simulink model "Propeller_Control_Prime_Mover"  (R2021b)
settings: Solver=VariableStepAuto  StartTime=0.0  StopTime=30.0  RelTol=1e-3
libraries: fl_lib x11, nesl_utility x4, slpidlib x2, ee_lib x1, sdl_lib x1
settings Model: Creator=Rishi  LastModifiedBy=Rishi

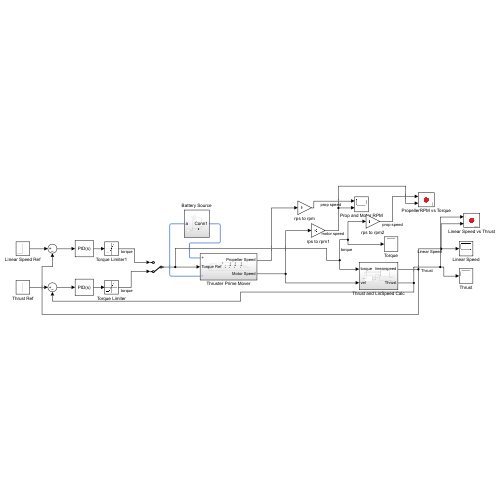
[thumbnail: Simulink's stored preview of the top-level diagram]
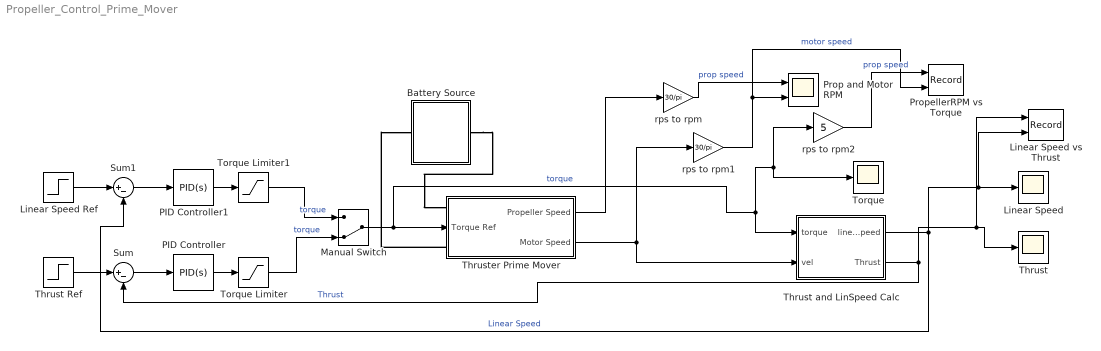
== system Propeller_Control_Prime_Mover ==
  Battery Source : Subsystem
  Linear Speed : Scope
  Linear Speed Ref : Step  After=3  SampleTime=0
  Linear Speed vs Thrust : Record  FileSettingsInternal="{\"entries\":[{\"content\":{\"excelSettings\":{\"content\":{},\"type\":\"Streamout.ExcelSettings\"}},\"type\":\"Streamout.FileSettingStorage\",\"uuid\":\"f38cdbd6-b5c5-4525-af82-986570d2f1bb\"}],\"packageUris\":[\"http://schema.mathworks.com/mf0/streamout_blocks/R2020a\"],\"version\":\"1.0\"}"  Layout=[1 1]  SignalsInternal="{\"entries\":[{\"content\":{\"signals\":[{\"content\":{\"blockPath\":[\"Propeller_Control_Prime_Mover/Linear Speed vs Thrust\"],\"channel\":[],\"dimensions\":[1],\"domain\":\"Propeller_Control_Prime_Mover/Linear Speed vs Thrust\",\"lineColor\":\"#a2142f\",\"plots\":[1],\"port\":1,\"sid\":[\"\"],\"signalID\":332,\"signalName\":\"Thrust\"},\"type\":\"RecordBlkView.Signal\",\"uuid\":\"575c3137-ab97-410f-b3d3-826d395c1239\"},{\"content\":{\"blockPath\":[\"Propeller_Control_Prime_Mover/Linear Speed vs Thrust\"],\"channel\":[],\"dimensions\":[1],\"domain\":\"Propeller_Control_Prime_Mover/Linear Speed vs Thrust\",\"lineColor\":\"#139fff\",\"plots\":[1],\"port\":2,\"sid\":[\"\"],\"signalID\":336,\"signalName\":\"Linear Speed\"},\"type\":\"RecordBlkView.Signal\",\"uuid\":\"f93925d7-110e-4419-9b3e-40073e6103b4\"}]},\"type\":\"RecordBlkView.InputSignals\",\"uuid\":\"601741f8-a10c-45ed-a42c-22fcf3854612\"}],\"packageUris\":[\"http://schema.mathworks.com/mf0/streamout_blocks/R2020a\"],\"version\":\"1.0\"}"  VisualizationBindings="{\"xyplotplugin\":{\"info\":[{\"series\":[{\"bindingParametersList\":[{\"parameter\":\"X-Axis\",\"signalID\":332,\"signalName\":\"Thrust\"},{\"parameter\":\"Y-Axis\",\"signalID\":336,\"signalName\":\"Linear Speed\"}],\"seriesID\":64183}],\"subplotID\":1}]}}"  CompatibilityTag=XY
  Manual Switch : ManualSwitch  CurrentSetting=0
  PID Controller : slpidlib/PID Controller  Controller=PID  Form=Parallel  TimeDomain=Continuous-time  UseExternalTs=off  SampleTime=-1  IntegratorMethod=Forward Euler  FilterMethod=Forward Euler  ControllerParametersSource=internal  P=0.0808899689686358  I=0.058736929683079  D=-0.00606531904447916  UseFilter=on  N=1.40895966466238  TunerSelectOption=Transfer Function Based (PID Tuner App)  InitialConditionSource=internal  InitialConditionForIntegrator=0  InitialConditionForFilter=0  DifferentiatorICPrevScaledInput=0  ExternalReset=none  TrackingMode=off  Kt=1  LimitOutput=off  SatLimitsSource=internal  UpperSaturationLimit=inf  LowerSaturationLimit=-inf  LinearizeAsGain=on  AntiWindupMode=none  Kb=1  POutMin=[]  POutMax=[]  IOutMin=[]  IOutMax=[]  DOutMin=[]  DOutMax=[]  NOutMin=[]  NOutMax=[]  SumOutMin=[]  SumOutMax=[]  SaturationOutMin=[]  SaturationOutMax=[]  PParamMin=[]  PParamMax=[]  IParamMin=[]  IParamMax=[]  DParamMin=[]  DParamMax=[]  NParamMin=[]  NParamMax=[]  KbParamMin=[]  KbParamMax=[]  KtParamMin=[]  KtParamMax=[]  KbOutMin=[]  KbOutMax=[]  KtOutMin=[]  KtOutMax=[]  IntegratorOutMin=[]  IntegratorOutMax=[]  FilterOutMin=[]  FilterOutMax=[]  SumI1OutMin=[]  SumI1OutMax=[]  SumI2OutMin=[]  SumI2OutMax=[]  SumI3OutMin=[]  SumI3OutMax=[]  SumI4OutMin=[]  SumI4OutMax=[]  SumDOutMin=[]  SumDOutMax=[]  DifferentiatorOutMin=[]  DifferentiatorOutMax=[]  FilterDiffOutCoefMin=[]  FilterDiffOutCoefMax=[]  ReciprocalOutMin=[]  ReciprocalOutMax=[]  SumDenOutMin=[]  SumDenOutMax=[]  SumNumOutMin=[]  SumNumOutMax=[]  DivideOutMin=[]  DivideOutMax=[]  UdiffTsProdOutMin=[]  UdiffTsProdOutMax=[]  NTsProdOutMin=[]  NTsProdOutMax=[]  UintegralTsProdOutMin=[]  UintegralTsProdOutMax=[]  UngainTsProdOutMin=[]  UngainTsProdOutMax=[]  IntegratorContinuousStateAttributes=''  IntegratorStateMustResolveToSignalObject=off  IntegratorRTWStateStorageClass=Auto  FilterContinuousStateAttributes=''  FilterStateMustResolveToSignalObject=off  FilterRTWStateStorageClass=Auto  ParallelPVariant=InternalParameters  IdealPVariant=Disabled  IVariant=InternalParameters  DVariant=InternalParameters  IntegratorVariant=Continuous  SatVariant=Disabled  AWVariant=Passthrough  PCopyVariant=Disabled  TRVariant=Disabled  FdbkBlocksVariant=Forward  IdealPFdbkVariant=Disabled  SatFdbkVariant=Disabled  DerivativeFilterVariant=ContFilter  NVariant=InternalParameters  NCopyVariant=Disabled  FilterICVariant=InternalICsFilter  IntegratorICVariant=InternalICs  ExternalResetVariant=Disabled  TRSumVariant=Passthrough  SumFdbkVariant=Disabled  SumVariant=Sum_PID  TsampFilterVariant=InternalTs  TsampNgainVariant=Passthrough  TsampIntegralVariant=Passthrough  ExternalSaturationOutDataTypeStr=Inherit: Same as second input
  PID Controller1 : slpidlib/PID Controller  Controller=PID  Form=Parallel  TimeDomain=Continuous-time  UseExternalTs=off  SampleTime=-1  IntegratorMethod=Forward Euler  FilterMethod=Forward Euler  ControllerParametersSource=internal  P=0  I=0.957539779346888  D=0  UseFilter=on  N=100  TunerSelectOption=Transfer Function Based (PID Tuner App)  InitialConditionSource=internal  InitialConditionForIntegrator=0  InitialConditionForFilter=0  DifferentiatorICPrevScaledInput=0  ExternalReset=none  TrackingMode=off  Kt=1  LimitOutput=off  SatLimitsSource=internal  UpperSaturationLimit=inf  LowerSaturationLimit=-inf  LinearizeAsGain=on  AntiWindupMode=none  Kb=1  POutMin=[]  POutMax=[]  IOutMin=[]  IOutMax=[]  DOutMin=[]  DOutMax=[]  NOutMin=[]  NOutMax=[]  SumOutMin=[]  SumOutMax=[]  SaturationOutMin=[]  SaturationOutMax=[]  PParamMin=[]  PParamMax=[]  IParamMin=[]  IParamMax=[]  DParamMin=[]  DParamMax=[]  NParamMin=[]  NParamMax=[]  KbParamMin=[]  KbParamMax=[]  KtParamMin=[]  KtParamMax=[]  KbOutMin=[]  KbOutMax=[]  KtOutMin=[]  KtOutMax=[]  IntegratorOutMin=[]  IntegratorOutMax=[]  FilterOutMin=[]  FilterOutMax=[]  SumI1OutMin=[]  SumI1OutMax=[]  SumI2OutMin=[]  SumI2OutMax=[]  SumI3OutMin=[]  SumI3OutMax=[]  SumI4OutMin=[]  SumI4OutMax=[]  SumDOutMin=[]  SumDOutMax=[]  DifferentiatorOutMin=[]  DifferentiatorOutMax=[]  FilterDiffOutCoefMin=[]  FilterDiffOutCoefMax=[]  ReciprocalOutMin=[]  ReciprocalOutMax=[]  SumDenOutMin=[]  SumDenOutMax=[]  SumNumOutMin=[]  SumNumOutMax=[]  DivideOutMin=[]  DivideOutMax=[]  UdiffTsProdOutMin=[]  UdiffTsProdOutMax=[]  NTsProdOutMin=[]  NTsProdOutMax=[]  UintegralTsProdOutMin=[]  UintegralTsProdOutMax=[]  UngainTsProdOutMin=[]  UngainTsProdOutMax=[]  IntegratorContinuousStateAttributes=''  IntegratorStateMustResolveToSignalObject=off  IntegratorRTWStateStorageClass=Auto  FilterContinuousStateAttributes=''  FilterStateMustResolveToSignalObject=off  FilterRTWStateStorageClass=Auto  ParallelPVariant=InternalParameters  IdealPVariant=Disabled  IVariant=InternalParameters  DVariant=InternalParameters  IntegratorVariant=Continuous  SatVariant=Disabled  AWVariant=Passthrough  PCopyVariant=Disabled  TRVariant=Disabled  FdbkBlocksVariant=Forward  IdealPFdbkVariant=Disabled  SatFdbkVariant=Disabled  DerivativeFilterVariant=ContFilter  NVariant=InternalParameters  NCopyVariant=Disabled  FilterICVariant=InternalICsFilter  IntegratorICVariant=InternalICs  ExternalResetVariant=Disabled  TRSumVariant=Passthrough  SumFdbkVariant=Disabled  SumVariant=Sum_PID  TsampFilterVariant=InternalTs  TsampNgainVariant=Passthrough  TsampIntegralVariant=Passthrough  ExternalSaturationOutDataTypeStr=Inherit: Same as second input
  Prop and Motor RPM : Scope  NumInputPorts=2
  PropellerRPM vs Torque : Record  FileSettingsInternal="{\"entries\":[{\"content\":{\"excelSettings\":{\"content\":{},\"type\":\"Streamout.ExcelSettings\"}},\"type\":\"Streamout.FileSettingStorage\",\"uuid\":\"e7f1eaa3-e328-4bb8-9999-0087dc1a7fd9\"}],\"packageUris\":[\"http://schema.mathworks.com/mf0/streamout_blocks/R2020a\"],\"version\":\"1.0\"}"  Layout=[1 1]  SignalsInternal="{\"entries\":[{\"content\":{\"signals\":[{\"content\":{\"blockPath\":[\"Propeller_Control_Prime_Mover/PropellerRPM vs Torque\"],\"channel\":[],\"dimensions\":[1],\"domain\":\"Propeller_Control_Prime_Mover/PropellerRPM vs Torque\",\"lineColor\":\"#64d413\",\"plots\":[],\"port\":1,\"sid\":[\"\"],\"signalID\":340,\"signalName\":\"prop speed\"},\"type\":\"RecordBlkView.Signal\",\"uuid\":\"83d94086-b276-4ada-afda-b43e66d6f884\"},{\"content\":{\"blockPath\":[\"Propeller_Control_Prime_Mover/PropellerRPM vs Torque\"],\"channel\":[],\"dimensions\":[1],\"domain\":\"Propeller_Control_Prime_Mover/PropellerRPM vs Torque\",\"lineColor\":\"#ff13a6\",\"plots\":[],\"port\":2,\"sid\":[\"\"],\"signalID\":344,\"signalName\":\"motor speed\"},\"type\":\"RecordBlkView.Signal\",\"uuid\":\"5dc8b065-5f7c-49e4-81b4-50af2d2f00db\"}]},\"type\":\"RecordBlkView.InputSignals\",\"uuid\":\"fe2e9c10-fa43-4037-ab47-88955eef5109\"}],\"packageUris\":[\"http://schema.mathworks.com/mf0/streamout_blocks/R2020a\"],\"version\":\"1.0\"}"  VisualizationBindings="{\"xyplotplugin\":{\"info\":[{\"series\":[{\"bindingParametersList\":[{\"parameter\":\"X-Axis\",\"signalID\":9,\"signalName\":\"prop speed\"},{\"parameter\":\"Y-Axis\",\"signalID\":12,\"signalName\":\"motor speed\"}],\"seriesID\":39395}],\"subplotID\":1}]}}"  CompatibilityTag=XY
  Sum : Sum  Inputs=|+-
  Sum1 : Sum  Inputs=|+-
  Thrust : Scope
  Thrust Ref : Step  After=98  SampleTime=0
  Thrust and LinSpeed Calc : Subsystem
  Thruster Prime Mover : Subsystem
      settings: PortSchema="{\"entries\":[{\"content\":{\"sides\":[{\"content\":{\"connectorIds\":[\"LConn1\",\"In1\",\"LConn2\"]},\"type\":\"ConnectorPlacement.EquallySpacedRectSide\",\"uuid\":\"b491ab2f-3c91-4c99-a87c-c51358079dd3\"},{\"content\":{\"connectorIds\":[\"Out1\",\"Out2\"],\"side\":\"RIGHT\"},\"type\":\"ConnectorPlacement.EquallySpacedRectSide\",\"uuid\":\"68efad03-1b86-4427-b220-44990910d7ff\"},{\"content\":{\"connectorIds\":[],\"side\":\"TOP\"},\"type\":\"ConnectorPlacement.EquallySpacedRectSide\",\"uuid\":\"6c75a4a0-8522-4b4f-a5fb-dcf7bbf55362\"}]},\"type\":\"ConnectorPlacement.EquallySpacedConnector\",\"uuid\":\"388c7d20-d64b-442d-a00b-569f4554c2be\"}],\"packageUris\":[\"http://schema.mathworks.com/mf0/Connector/R2020b\"],\"version\":\"1.0\"}"
  Torque : Scope
  Torque Limiter : Saturate  UpperLimit=5  LowerLimit=0
  Torque Limiter1 : Saturate  UpperLimit=5  LowerLimit=0
  rps to rpm : Gain  Gain=30/pi
  rps to rpm1 : Gain  Gain=30/pi
  rps to rpm2 : Gain  Gain=5
  wires:
  Thrust Ref/1 -> Sum/1
  Thruster Prime Mover/2(Motor Speed) -> rps to rpm1/1, Thrust and LinSpeed Calc/2(vel)
  Torque Limiter/1 -> Manual Switch/2  "torque"
  PID Controller/1 -> Torque Limiter/1
  Sum/1 -> PID Controller/1
  Thruster Prime Mover/1(Propeller Speed) -> rps to rpm/1
  Torque Limiter1/1 -> Manual Switch/1  "torque"
  PID Controller1/1 -> Torque Limiter1/1
  Linear Speed Ref/1 -> Sum1/1
  Sum1/1 -> PID Controller1/1
  Manual Switch/1 -> rps to rpm2/1, Torque/1, Thrust and LinSpeed Calc/1(torque), Thruster Prime Mover/1(Torque Ref)  "torque"
  Thrust and LinSpeed Calc/2(Thrust) -> Linear Speed vs Thrust/1, Thrust/1, Sum/2  "Thrust"
  Thrust and LinSpeed Calc/1(linearspeed) -> Linear Speed vs Thrust/2, Linear Speed/1, Sum1/2  "Linear Speed"
  rps to rpm/1 -> Prop and Motor RPM/1  "prop speed"
  rps to rpm1/1 -> PropellerRPM vs Torque/2, Prop and Motor RPM/2  "motor speed"
  rps to rpm2/1 -> PropellerRPM vs Torque/1  "prop speed"
  connections:
  Battery Source/LConn1 -- Thruster Prime Mover/LConn1
  Thruster Prime Mover/LConn2 -- Battery Source/RConn1

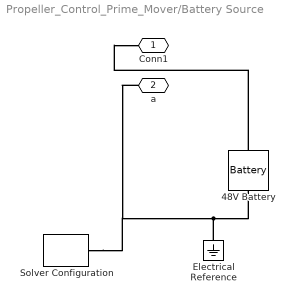
== system Propeller_Control_Prime_Mover/Battery Source ==
  48V Battery : ee_lib/Sources/Battery  Vnom=48 V  prm_dir=1  R1_dis=2 Ohm  R1_ch=2 Ohm  R1=2 Ohm  prm_AH=1  AH=50 A*hr  V1=11.5 V  AH1=25 A*hr  prm_R2=1  R2=2000 Ohm  prm_dyn=1  Rp1=0.005 Ohm  tau1=30 s  Rp2=0.005 Ohm  tau2=30 s  Rp3=0.005 Ohm  tau3=30 s  Rp4=0.005 Ohm  tau4=30 s  Rp5=0.005 Ohm  tau5=30 s  prm_fade=1  N_fade=100  AH_fade=45 A*hr  R1_fade=2.02 Ohm  R1_ch_fade=2.02 Ohm  V1_fade=10.35 V  prm_age=1  prm_age_OCV=1  OCV_age=0.9  SOC_age=60  delta_time_age_vec=[0] d  temperature_age_vec=[273] K  OCV_scaling_age=2.2134e6  OCV_offset_age=1.632e6  temp_exp_age=0.515833569 V  t_exp_age=0.75  i_specify=off  i_priority=None  i=0 A  i_nominal_specify=off  i_nominal_unit=A  i_nominal_value=1  v_specify=off  v_priority=None  v=0 V  v_nominal_specify=off  v_nominal_unit=V  v_nominal_value=1  charge_specify=off  charge_priority=High  charge=50 A*hr  charge_nominal_specify=off  charge_nominal_unit=A*hr  charge_nominal_value=1  num_cycles_specify=off  num_cycles_priority=High  num_cycles=0  num_cycles_nominal_specify=off  num_cycles_nominal_unit=1  num_cycles_nominal_value=1  Tmeas=298.15 K  Tmeas_age=298.15 K  Vnom_T2=12 V  R1_T2=2.2 Ohm  R1_T2_dis=2.2 Ohm  R1_T2_ch=2.2 Ohm  V1_T2=11.4 V  R2_T2=2200 Ohm  Rp1_T2=0.005 Ohm  tau1_T2=30 s  Rp2_T2=0.005 Ohm  tau2_T2=30 s  Rp3_T2=0.005 Ohm  tau3_T2=30 s  Rp4_T2=0.005 Ohm  tau4_T2=30 s  Rp5_T2=0.005 Ohm  tau5_T2=30 s  Tmeas2=273.15 K  thermal_mass=30000 J/K  temperature_specify=off  temperature_priority=High  temperature=298.15 K  temperature_nominal_specify=off  temperature_nominal_unit=K  temperature_nominal_value=1
  Electrical Reference : fl_lib/Electrical/Electrical Elements/Electrical Reference
  Solver Configuration : nesl_utility/Solver Configuration  PhysicalDomain=network_engine_domain  SubClassName=solver  LeftPortType=input  RightPortType=generic  Tones=[]  Harmonics=[]  SimulateNoise=off  Profile=off  UseLocalSampling=off  EnableSwitchedLinearOptims=on  FrequencyDomain=off  UseCCode=off  RelTol=0.001  AbsTol=1e-06  MinStep=1e-09  ToWorkspace=off  RevertToSquareIcSolve=off  NumHomotopyIterations=100  PhasorMode=off  PhasorModeNumHarmonics=1  DoDC=off  ResidualTolerance=1e-09  UseLocalSolver=off  LocalSolverChoice=NE_BACKWARD_EULER_ADVANCER  LocalSolverSampleTime=0.001  DoFixedCost=off  MaxNonlinIter=3  MaxModeIter=2  ComputeImpulses=off  ImpulseIterations=2  LinearAlgebra=auto  EquationFormulation=NE_TIME_EF  DelaysMemoryBudget=1024  AutomaticFiltering=on  FilteringTimeConstant=0.001  PartitionStorageMethod=AS_NEEDED  PartitionMemoryBudget=1024  PartitionMethod=ROBUST
      settings: SourceProductBaseCode=PW,SS
  Conn1 : PMIOPort  Side=Left
  a : PMIOPort  Port=2  Side=Right
  connections:
  Electrical Reference/LConn1 -- 48V Battery/RConn1 -- a/RConn1 -- Solver Configuration/RConn1
  48V Battery/LConn1 -- Conn1/RConn1

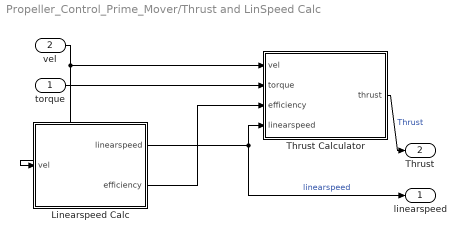
== system Propeller_Control_Prime_Mover/Thrust and LinSpeed Calc ==
  torque : Inport
  vel : Inport  Port=2
  Linearspeed Calc : MATLAB Function  TreatAsAtomicUnit=on
  Thrust Calculator : MATLAB Function  TreatAsAtomicUnit=on
  linearspeed : Outport
  Thrust : Outport  Port=2
  wires:
  vel/1 -> Linearspeed Calc/1(vel), Thrust Calculator/1(vel)
  torque/1 -> Thrust Calculator/2(torque)
  Thrust Calculator/1(thrust) -> Thrust/1  "Thrust"
  Linearspeed Calc/1(linearspeed) -> linearspeed/1, Thrust Calculator/4(linearspeed)  "linearspeed"
  Linearspeed Calc/2(efficiency) -> Thrust Calculator/3(efficiency)

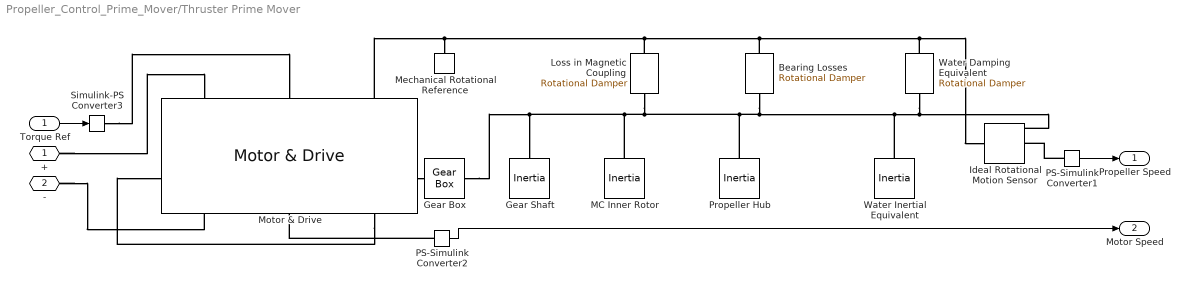
== system Propeller_Control_Prime_Mover/Thruster Prime Mover ==
  Torque Ref : Inport
  Bearing Losses : fl_lib/Mechanical/Rotational Elements/Rotational Damper  D=0.01 N*m/(rad/s)  w_specify=off  w_priority=None  w=0 rad/s  w_nominal_specify=off  w_nominal_unit=rad/s  w_nominal_value=1  t_specify=off  t_priority=None  t=0 N*m  t_nominal_specify=off  t_nominal_unit=N*m  t_nominal_value=1
  Gear Box : fl_lib/Mechanical/Mechanisms/Gear Box  ratio=5  t_in_specify=off  t_in_priority=None  t_in=0 N*m  t_in_nominal_specify=off  t_in_nominal_unit=N*m  t_in_nominal_value=1  t_out_specify=off  t_out_priority=None  t_out=0 N*m  t_out_nominal_specify=off  t_out_nominal_unit=N*m  t_out_nominal_value=1
  Gear Shaft : fl_lib/Mechanical/Rotational Elements/Inertia  inertia=6.525e-08 kg*m^2  num_ports=foundation.enum.numPorts2.one  w_specify=off  w_priority=High  w=0 rad/s  w_nominal_specify=off  w_nominal_unit=rad/s  w_nominal_value=1  t_specify=off  t_priority=None  t=0 N*m  t_nominal_specify=off  t_nominal_unit=N*m  t_nominal_value=1
  Ideal Rotational Motion Sensor : fl_lib/Mechanical/Mechanical Sensors/Ideal Rotational Motion Sensor  wrap_angle=simscape.enum.onoff.off  offset=0 rad
  Loss in Magnetic Coupling : fl_lib/Mechanical/Rotational Elements/Rotational Damper  D=0.001 N*m*s/rad  w_specify=off  w_priority=None  w=0 rad/s  w_nominal_specify=off  w_nominal_unit=rad/s  w_nominal_value=1  t_specify=off  t_priority=None  t=0 N*m  t_nominal_specify=off  t_nominal_unit=N*m  t_nominal_value=1
  MC Inner Rotor : fl_lib/Mechanical/Rotational Elements/Inertia  inertia=0.000145 kg*m^2  num_ports=foundation.enum.numPorts2.one  w_specify=off  w_priority=High  w=0 rad/s  w_nominal_specify=off  w_nominal_unit=rad/s  w_nominal_value=1  t_specify=off  t_priority=None  t=0 N*m  t_nominal_specify=off  t_nominal_unit=N*m  t_nominal_value=1
  Mechanical Rotational Reference : fl_lib/Mechanical/Rotational Elements/Mechanical Rotational Reference
  Motor & Drive : sdl_lib/Engines & Motors/Motor & Drive  torque_max=5 N*m  power_max=0.8 kW  Tc=0.02 s  eff=90  w_eff=2500 rpm  T_eff=3 N*m  thermal_port=simscape.enum.thermaleffects.omit  thermal_mass=100 J/K  temperature_specify=off  temperature_priority=High  temperature=300 K  temperature_nominal_specify=off  temperature_nominal_unit=K  temperature_nominal_value=1
      settings: SourceProductBaseCode=LD  InternalSimscapePortConfiguration="{\"Bottom\":[],\"Left\":[{\"id\":\"Vp\",\"label\":\"+\",\"type\":\"foundation.electrical.electrical\"},{\"id\":\"Tr\",\"label\":\"Tr\",\"type\":\"input\"},{\"id\":\"R\",\"label\":\"R\",\"type\":\"foundation.mechanical.rotational.rotational\"}],\"Right\":[{\"id\":\"Vm\",\"label\":\"-\",\"type\":\"foundation.electrical.electrical\"},{\"id\":\"Omega\",\"label\":\"w\",\"type\":\"output\"},{\"id\":\"C\",\"label\":\"C\",\"type\":\"foundation.mechanical.rotational.rotational\"}],\"Top\":[]}"
  PS-Simulink Converter1 : nesl_utility/PS-Simulink Converter  PhysicalDomain=network_engine_domain  SubClassName=ps_output  LeftPortType=input  RightPortType=output  PseudoPeriodic=off  Frequencies=[]  Unit=inherit  AffineConversion=off
      settings: SourceProductBaseCode=PW,SS
  PS-Simulink Converter2 : nesl_utility/PS-Simulink Converter  PhysicalDomain=network_engine_domain  SubClassName=ps_output  LeftPortType=input  RightPortType=output  PseudoPeriodic=off  Frequencies=[]  Unit=inherit  AffineConversion=off
      settings: SourceProductBaseCode=PW,SS
  Propeller Hub : fl_lib/Mechanical/Rotational Elements/Inertia  inertia=0.02398 kg*m^2  num_ports=foundation.enum.numPorts2.one  w_specify=off  w_priority=High  w=0 rad/s  w_nominal_specify=off  w_nominal_unit=rad/s  w_nominal_value=1  t_specify=off  t_priority=None  t=0 N*m  t_nominal_specify=off  t_nominal_unit=N*m  t_nominal_value=1
  Simulink-PS Converter3 : nesl_utility/Simulink-PS Converter  PhysicalDomain=network_engine_domain  SubClassName=ps_input  LeftPortType=input  RightPortType=output  PseudoPeriodic=off  Frequencies=[]  NoiseDistribution=none  NoiseParameters=[]  Unit=1  AffineConversion=off  FilteringAndDerivatives=provide  SimscapeFilterOrder=1  InputFilterTimeConstant=0.001  UdotUserProvided=0
      settings: SourceProductBaseCode=PW,SS
  Water Damping Equivalent : fl_lib/Mechanical/Rotational Elements/Rotational Damper  D=1.1 N*m/(rad/s)  w_specify=off  w_priority=None  w=0 rad/s  w_nominal_specify=off  w_nominal_unit=rad/s  w_nominal_value=1  t_specify=off  t_priority=None  t=0 N*m  t_nominal_specify=off  t_nominal_unit=N*m  t_nominal_value=1
  Water Inertial Equivalent : fl_lib/Mechanical/Rotational Elements/Inertia  inertia=0.08 kg*m^2  num_ports=foundation.enum.numPorts2.one  w_specify=off  w_priority=High  w=0 rad/s  w_nominal_specify=off  w_nominal_unit=rad/s  w_nominal_value=1  t_specify=off  t_priority=None  t=0 N*m  t_nominal_specify=off  t_nominal_unit=N*m  t_nominal_value=1
  + : PMIOPort  Side=Left
  - : PMIOPort  Port=2  Side=Left
  Propeller Speed : Outport
  Motor Speed : Outport  Port=2
  wires:
  PS-Simulink Converter1/1 -> Propeller Speed/1
  Torque Ref/1 -> Simulink-PS Converter3/1
  PS-Simulink Converter2/1 -> Motor Speed/1
  connections:
  -/RConn1 -- Motor & Drive/RConn1
  +/RConn1 -- Motor & Drive/LConn1
  Gear Box/RConn1 -- Bearing Losses/RConn1 -- Water Inertial Equivalent/LConn1 -- Water Damping Equivalent/RConn1 -- Ideal Rotational Motion Sensor/RConn1 -- Propeller Hub/LConn1 -- Loss in Magnetic Coupling/RConn1 -- MC Inner Rotor/LConn1 -- Gear Shaft/LConn1
  Motor & Drive/LConn3 -- Loss in Magnetic Coupling/LConn1 -- Bearing Losses/LConn1 -- Water Damping Equivalent/LConn1 -- Ideal Rotational Motion Sensor/LConn1 -- Mechanical Rotational Reference/LConn1
  Motor & Drive/RConn3 -- Gear Box/LConn1
  PS-Simulink Converter1/LConn1 -- Ideal Rotational Motion Sensor/RConn2
  Simulink-PS Converter3/RConn1 -- Motor & Drive/LConn2
  PS-Simulink Converter2/LConn1 -- Motor & Drive/RConn2

== matlab function Propeller_Control_Prime_Mover/Thrust and LinSpeed Calc/Linearspeed Calc ==
  data: vel input; linearspeed output; efficiency output
function [linearspeed,efficiency] = fcn(vel)
pitch_angle= 27;
prop_d=0.35;
pitch= tand(pitch_angle)*prop_d*pi;
rpm=vel*30/pi;
if(rpm<10)
    efficiency=0.1;
elseif(rpm<20)
    efficiency=0.2;
elseif(rpm<30)
    efficiency=0.3; 
elseif(rpm<40)
    efficiency=0.4;
elseif(rpm<50)
    efficiency=0.5;
elseif(rpm<100)
    efficiency=0.6;
else
    efficiency=0.7;
end
linearspeed=pitch*efficiency*rpm/60;
end

== matlab function Propeller_Control_Prime_Mover/Thrust and LinSpeed Calc/Thrust Calculator ==
  data: vel input; thrust output; torque input; efficiency input; linearspeed input
function thrust = fcn(vel, torque,efficiency,linearspeed)
thrust=vel*torque*efficiency/0.1+linearspeed;
end
